simulink model "yidongshi"  (R2025b)
settings: Solver=VariableStepAuto  StartTime=0.0  StopTime=65  RelTol=1e-3
values from neighbouring files (symbols this model uses):
  ADAMS_cwd = 'D:\2022110616\yidongshi'    [Controls_Plant_1.m]
  ADAMS_exec = ''    [Controls_Plant_1.m]
  ADAMS_host = 'yangyuheng701'    [Controls_Plant_1.m]
  ADAMS_init = ''    [Controls_Plant_1.m]
  ADAMS_inputs = 'INT_YOU!INT_ZUO!INV_SHENGJIANG!INV_SHENSUO!INV_XUANZHUAN!TURN'    [Controls_Plant_1.m]
  ADAMS_outputs = 'OUT_CMX!OUT_CMY!OUT_CMZ!OUT_SHENGJIANG!OUT_SHENSUO!OUT_V_YOU!OUT_V_ZUO!OUT_XUANZHUAN!ZHUSHUI_X!ZHUSHUI_Y!ZHUSHUI_Z'    [Controls_Plant_1.m]
  ADAMS_prefix = 'Controls_Plant_1'    [Controls_Plant_1.m]
  ADAMS_static = 'no'    [Controls_Plant_1.m]
  ADAMS_sysdir = 'D:\adams\'    [Controls_Plant_1.m]
libraries: slpidlib x2
settings Model: Creator=yangy  LastModifiedBy=yangy

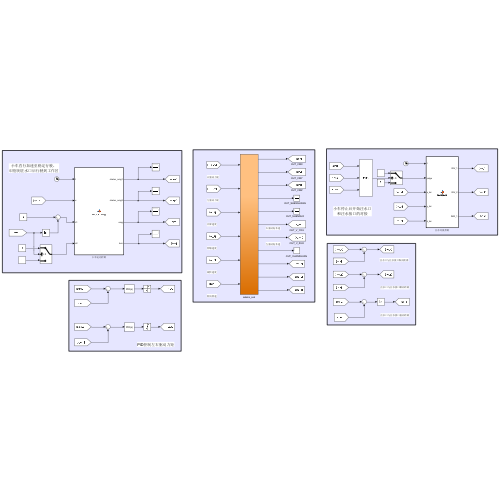
[thumbnail: Simulink's stored preview of the top-level diagram]
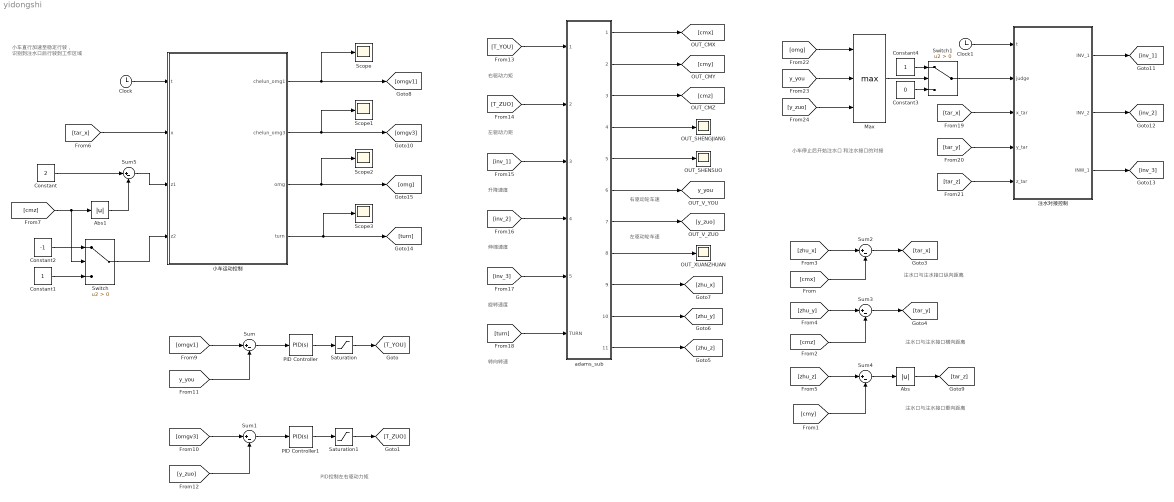
== system yidongshi ==
  note: PID控制左右驱动力矩
  note: 注水口与注水接口纵向距离
  note: 注水口与注水接口横向距离
  note: 注水口与注水接口垂向距离
  note: 小车停止后开始注水口
      | 和注水接口的对接
  note: 小车直行加速至稳定行驶，
      | 识别到注水口后行驶到工作区域
  note: 右驱动力矩
  note: 左驱动力矩
  note: 升降速度
  note: 伸缩速度
  note: 旋转速度
  note: 转向转速
  note: 右驱动轮车速
  note: 左驱动轮车速
  Abs : Abs  SaturateOnIntegerOverflow=off
  Abs1 : Abs  SaturateOnIntegerOverflow=off
  Clock : Clock
  Clock1 : Clock
  Constant : Constant  Value=2
  Constant1 : Constant
  Constant2 : Constant  Value=-1
  Constant3 : Constant  Value=0
  Constant4 : Constant
  Max : MinMax  Function=max  Inputs=3
  "OUT_SHENGJIANG     " : Scope
      settings: DataLoggingVariableName=ScopeData6
  "OUT_SHENSUO     " : Scope
      settings: DataLoggingVariableName=ScopeData7
  "OUT_XUANZHUAN " : Scope
      settings: DataLoggingVariableName=ScopeData8
  PID Controller : slpidlib/PID Controller  Controller=PID  Form=Parallel  TimeDomain=Continuous-time  UseExternalTs=off  SampleTime=-1  IntegratorMethod=Forward Euler  FilterMethod=Forward Euler  ControllerParametersSource=internal  P=1.7  I=0.1  UseKiTs=off  D=0.1  UseExternalDerivativeSource=off  N=100  UseFilter=on  TunerSelectOption=Transfer Function Based (PID Tuner App)  InitialConditionSource=internal  InitialConditionForIntegrator=0  InitialConditionForFilter=0  DifferentiatorICPrevScaledInput=0  ExternalReset=none  TrackingMode=off  Kt=1  LimitOutput=off  SatLimitsSource=internal  UpperSaturationLimit=inf  LowerSaturationLimit=-inf  LinearizeAsGain=on  AntiWindupMode=none  Kb=1  LimitIntegrator=off  UpperIntegratorSaturationLimit=inf  LowerIntegratorSaturationLimit=-inf  POutMin=[]  POutMax=[]  IOutMin=[]  IOutMax=[]  DOutMin=[]  DOutMax=[]  NOutMin=[]  NOutMax=[]  SumOutMin=[]  SumOutMax=[]  SaturationOutMin=[]  SaturationOutMax=[]  PParamMin=[]  PParamMax=[]  IParamMin=[]  IParamMax=[]  DParamMin=[]  DParamMax=[]  NParamMin=[]  NParamMax=[]  KbParamMin=[]  KbParamMax=[]  KtParamMin=[]  KtParamMax=[]  KbOutMin=[]  KbOutMax=[]  KtOutMin=[]  KtOutMax=[]  IntegratorOutMin=[]  IntegratorOutMax=[]  FilterOutMin=[]  FilterOutMax=[]  SumI1OutMin=[]  SumI1OutMax=[]  SumI2OutMin=[]  SumI2OutMax=[]  SumI3OutMin=[]  SumI3OutMax=[]  SumI4OutMin=[]  SumI4OutMax=[]  SumDOutMin=[]  SumDOutMax=[]  DifferentiatorOutMin=[]  DifferentiatorOutMax=[]  FilterDiffOutCoefMin=[]  FilterDiffOutCoefMax=[]  ReciprocalOutMin=[]  ReciprocalOutMax=[]  SumDenOutMin=[]  SumDenOutMax=[]  SumNumOutMin=[]  SumNumOutMax=[]  DivideOutMin=[]  DivideOutMax=[]  UdiffTsProdOutMin=[]  UdiffTsProdOutMax=[]  NTsProdOutMin=[]  NTsProdOutMax=[]  UintegralTsProdOutMin=[]  UintegralTsProdOutMax=[]  UngainTsProdOutMin=[]  UngainTsProdOutMax=[]  ClampingZeroOutDataTypeStr=Inherit: Inherit via back propagation  ClampingZeroOutMin=[]  ClampingZeroOutMax=[]  FilterDenConstantOutDataTypeStr=Inherit: Inherit via back propagation  FilterDenConstantOutMin=[]  FilterDenConstantOutMax=[]  PCopyOutDataTypeStr=Inherit: Inherit via back propagation  PCopyOutMin=[]  PCopyOutMax=[]  NCopyOutDataTypeStr=Inherit: Inherit via back propagation  NCopyOutMin=[]  NCopyOutMax=[]  IntegratorContinuousStateAttributes=''  IntegratorStateMustResolveToSignalObject=off  IntegratorRTWStateStorageClass=Auto  FilterContinuousStateAttributes=''  FilterStateMustResolveToSignalObject=off  FilterRTWStateStorageClass=Auto  ParallelPVariant=InternalParameters  IdealPVariant=Disabled  IVariant=InternalParameters  DVariant=InternalParameters  IntegratorVariant=Continuous  SatVariant=Disabled  AWVariant=Passthrough  PCopyVariant=Disabled  TRVariant=Disabled  FdbkBlocksVariant=Forward  IdealPFdbkVariant=Disabled  SatFdbkVariant=Disabled  DerivativeFilterVariant=ContFilter  NVariant=InternalParameters  NCopyVariant=Disabled  FilterICVariant=InternalICsFilter  IntegratorICVariant=InternalICs  ExternalResetVariant=Disabled  TRSumVariant=Passthrough  SumFdbkVariant=Disabled  SumVariant=Sum_PID  TsampFilterVariant=InternalTs  TsampNgainVariant=Passthrough  TsampIntegralVariant=Disabled_SignalSpec  ExternalSaturationOutDataTypeStr=Inherit: Same as second input  DerivativeSourceVariant=ErrorSignal  PreIntVariant=InternalPreInt
  PID Controller1 : slpidlib/PID Controller  Controller=PID  Form=Parallel  TimeDomain=Continuous-time  UseExternalTs=off  SampleTime=-1  IntegratorMethod=Forward Euler  FilterMethod=Forward Euler  ControllerParametersSource=internal  P=1.7  I=0.1  UseKiTs=off  D=0.1  UseExternalDerivativeSource=off  N=100  UseFilter=on  TunerSelectOption=Transfer Function Based (PID Tuner App)  InitialConditionSource=internal  InitialConditionForIntegrator=0  InitialConditionForFilter=0  DifferentiatorICPrevScaledInput=0  ExternalReset=none  TrackingMode=off  Kt=1  LimitOutput=off  SatLimitsSource=internal  UpperSaturationLimit=inf  LowerSaturationLimit=-inf  LinearizeAsGain=on  AntiWindupMode=none  Kb=1  LimitIntegrator=off  UpperIntegratorSaturationLimit=inf  LowerIntegratorSaturationLimit=-inf  POutMin=[]  POutMax=[]  IOutMin=[]  IOutMax=[]  DOutMin=[]  DOutMax=[]  NOutMin=[]  NOutMax=[]  SumOutMin=[]  SumOutMax=[]  SaturationOutMin=[]  SaturationOutMax=[]  PParamMin=[]  PParamMax=[]  IParamMin=[]  IParamMax=[]  DParamMin=[]  DParamMax=[]  NParamMin=[]  NParamMax=[]  KbParamMin=[]  KbParamMax=[]  KtParamMin=[]  KtParamMax=[]  KbOutMin=[]  KbOutMax=[]  KtOutMin=[]  KtOutMax=[]  IntegratorOutMin=[]  IntegratorOutMax=[]  FilterOutMin=[]  FilterOutMax=[]  SumI1OutMin=[]  SumI1OutMax=[]  SumI2OutMin=[]  SumI2OutMax=[]  SumI3OutMin=[]  SumI3OutMax=[]  SumI4OutMin=[]  SumI4OutMax=[]  SumDOutMin=[]  SumDOutMax=[]  DifferentiatorOutMin=[]  DifferentiatorOutMax=[]  FilterDiffOutCoefMin=[]  FilterDiffOutCoefMax=[]  ReciprocalOutMin=[]  ReciprocalOutMax=[]  SumDenOutMin=[]  SumDenOutMax=[]  SumNumOutMin=[]  SumNumOutMax=[]  DivideOutMin=[]  DivideOutMax=[]  UdiffTsProdOutMin=[]  UdiffTsProdOutMax=[]  NTsProdOutMin=[]  NTsProdOutMax=[]  UintegralTsProdOutMin=[]  UintegralTsProdOutMax=[]  UngainTsProdOutMin=[]  UngainTsProdOutMax=[]  ClampingZeroOutDataTypeStr=Inherit: Inherit via back propagation  ClampingZeroOutMin=[]  ClampingZeroOutMax=[]  FilterDenConstantOutDataTypeStr=Inherit: Inherit via back propagation  FilterDenConstantOutMin=[]  FilterDenConstantOutMax=[]  PCopyOutDataTypeStr=Inherit: Inherit via back propagation  PCopyOutMin=[]  PCopyOutMax=[]  NCopyOutDataTypeStr=Inherit: Inherit via back propagation  NCopyOutMin=[]  NCopyOutMax=[]  IntegratorContinuousStateAttributes=''  IntegratorStateMustResolveToSignalObject=off  IntegratorRTWStateStorageClass=Auto  FilterContinuousStateAttributes=''  FilterStateMustResolveToSignalObject=off  FilterRTWStateStorageClass=Auto  ParallelPVariant=InternalParameters  IdealPVariant=Disabled  IVariant=InternalParameters  DVariant=InternalParameters  IntegratorVariant=Continuous  SatVariant=Disabled  AWVariant=Passthrough  PCopyVariant=Disabled  TRVariant=Disabled  FdbkBlocksVariant=Forward  IdealPFdbkVariant=Disabled  SatFdbkVariant=Disabled  DerivativeFilterVariant=ContFilter  NVariant=InternalParameters  NCopyVariant=Disabled  FilterICVariant=InternalICsFilter  IntegratorICVariant=InternalICs  ExternalResetVariant=Disabled  TRSumVariant=Passthrough  SumFdbkVariant=Disabled  SumVariant=Sum_PID  TsampFilterVariant=InternalTs  TsampNgainVariant=Passthrough  TsampIntegralVariant=Disabled_SignalSpec  ExternalSaturationOutDataTypeStr=Inherit: Same as second input  DerivativeSourceVariant=ErrorSignal  PreIntVariant=InternalPreInt
  Saturation : Saturate  UpperLimit=100  LowerLimit=-100
  Saturation1 : Saturate  UpperLimit=100  LowerLimit=-100
  Scope{,1..3} (4 alike) : Scope
      Scope settings: DataLoggingVariableName=ScopeData11
      Scope2 settings: DataLoggingVariableName=ScopeData2
  Sum{,1..5} (6 alike) : Sum  Inputs=|+-
  Switch : Switch  Criteria=u2 > Threshold  SaturateOnIntegerOverflow=off  InputSameDT=off
  Switch1 : Switch  Criteria=u2 > Threshold  SaturateOnIntegerOverflow=off  InputSameDT=off
  adams_sub : Subsystem
  小车运动控制 : MATLAB Function  TreatAsAtomicUnit=on
  注水对接控制 : MATLAB Function  TreatAsAtomicUnit=on
  tag scope: y_you=global
  wires:
  Clock/1 -> 小车运动控制/1(t)
  小车运动控制/1(chelun_omg1) -> Scope/1, [omgv1]
  小车运动控制/2(chelun_omg3) -> Scope1/1, [omgv3]
  Sum/1 -> PID Controller/1
  PID Controller/1 -> Saturation/1
  Saturation/1 -> [T_YOU]
  PID Controller1/1 -> Saturation1/1
  Saturation1/1 -> [T_ZUO]
  Sum1/1 -> PID Controller1/1
  [zhu_x] -> Sum2/1
  [cmx] -> Sum2/2
  [zhu_y] -> Sum3/1
  [cmz] -> Sum3/2
  [zhu_z] -> Sum4/1
  [cmy] -> Sum4/2
  Sum4/1 -> Abs/1
  Sum2/1 -> [tar_x]
  Sum3/1 -> [tar_y]
  Abs/1 -> [tar_z]
  [tar_x] -> 小车运动控制/2(x)
  Constant/1 -> Sum5/1
  Abs1/1 -> Sum5/2
  Sum5/1 -> 小车运动控制/3(z1)
  Constant2/1 -> Switch/1
  Constant1/1 -> Switch/3
  Switch/1 -> 小车运动控制/4(z2)
  [omgv1] -> Sum/1
  [y_you] -> Sum/2
  [omgv3] -> Sum1/1
  [y_zuo] -> Sum1/2
  小车运动控制/3(omg) -> Scope2/1, [omg]
  [cmz] -> Abs1/1, Switch/2
  小车运动控制/4(turn) -> Scope3/1, [turn]
  Constant3/1 -> Switch1/3
  [T_YOU] -> adams_sub/1("INT_YOU       ")
  [T_ZUO] -> adams_sub/2("INT_ZUO       ")
  [inv_1] -> adams_sub/3(INV_SHENGJIANG)
  [inv_3] -> adams_sub/5("INV_XUANZHUAN ")
  [turn] -> adams_sub/6("TURN          ")
  adams_sub/1("OUT_CMX       ") -> [cmx]
  adams_sub/2("OUT_CMY       ") -> [cmy]
  adams_sub/3("OUT_CMZ       ") -> [cmz]
  adams_sub/4(OUT_SHENGJIANG) -> "OUT_SHENGJIANG     "/1
  adams_sub/5("OUT_SHENSUO   ") -> "OUT_SHENSUO     "/1
  adams_sub/6("OUT_V_YOU     ") -> [y_you]
  adams_sub/7("OUT_V_ZUO     ") -> [y_zuo]
  [inv_2] -> adams_sub/4("INV_SHENSUO   ")
  adams_sub/8("OUT_XUANZHUAN ") -> "OUT_XUANZHUAN "/1
  adams_sub/9("ZHUSHUI_X     ") -> [zhu_x]
  adams_sub/10("ZHUSHUI_Y     ") -> [zhu_y]
  adams_sub/11("ZHUSHUI_Z     ") -> [zhu_z]
  [omg] -> Max/1
  [y_you] -> Max/2
  [y_zuo] -> Max/3
  Constant4/1 -> Switch1/1
  Max/1 -> Switch1/2
  [tar_z] -> 注水对接控制/5(z_tar)
  [tar_y] -> 注水对接控制/4(y_tar)
  [tar_x] -> 注水对接控制/3(x_tar)
  Switch1/1 -> 注水对接控制/2(judge)
  Clock1/1 -> 注水对接控制/1(t)
  注水对接控制/1(INV_1) -> [inv_1]
  注水对接控制/2(INV_2) -> [inv_2]
  注水对接控制/3(INW_1) -> [inv_3]

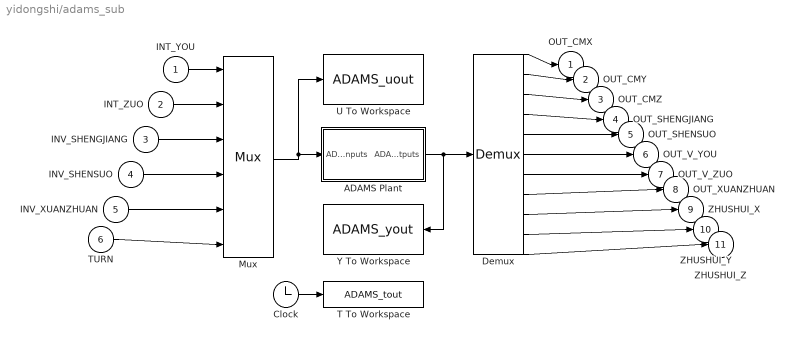
== system yidongshi/adams_sub ==
  "INT_YOU       " : Inport
  "INT_ZUO       " : Inport  Port=2
  INV_SHENGJIANG : Inport  Port=3
  "INV_SHENSUO   " : Inport  Port=4
  "INV_XUANZHUAN " : Inport  Port=5
  "TURN          " : Inport  Port=6
  ADAMS Plant : Subsystem  LoadFcn=|  InitFcn=clear mex  mask(Adams Plant){exevie=ADAMS_sysdir, nam_in=ADAMS_inputs, namout=ADAMS_outputs, nampre=ADAMS_prefix, outfil=ADAMS_prefix, exesol=ADAMS_exec, stat=ADAMS_static, inicmd=[ADAMS_init], exetyp=C++, comtyp=PIPE(DDE), workdir=ADAMS_cwd, ada_host=ADAMS_host, modani=batch, modsim=discrete, dft=no, simulink_lead_cosim=yes, pin_interp_order=0, pout_extrap_order=0, pin_extrap_order=0, pout_interp_order=0, dt_out=0.005, o_rate=1, more=off}
      | %check based on dialog box setting for when setting by popup menu                                             
      | if exist('ADAMS_solver_type')                                                                                 
      |   if strcmp(ADAMS_solver_type,'C++')                                                                          
      |     set_param(gcb,'exetyp','C++');                                                                            
      |   else                                                                                                        
      |     set_param(gcb,'exetyp','Fortran');                                                                        
      |   end                                                                                                         
      | else                                                                                                          
      |   set_param(gcb,'exetyp','C++');                                                                              
      | end                                                                                                           
      | %set the mode if using acar_solver                                                                            
      | %REQUIRED HERE BECAUSE BELOW CAUSES MDLTERMINATE TO BE CALLED 2 TIMES IN MIDDLE OF SIMULATION WHEN SET IN MASK
      |                                                                                                               
      | %enable the direct feedthrough, sim mode, anim mode parameters by default                                     
      |                                                                                                               
      | if exist('set_some_params_states')                                                                            
      |                                                                                                               
      |   set_some_params_states({'dft','modsim','modani'},{'on','on','on'},'MaskEnables',gcb)                        
      |   %turn on direct feedthrough option                                                                          
      |   set_some_params_states({'dft'},{'on'},'MaskVisibilities',gcb)                                               
      |                                                                                                               
      |  end                                                                                                          
      |                                                                                                               
      |                                                                                                               
      | if exist('ADAMS_exec')                                                                                        
      |   if and(strcmp(get_param(gcb,'exesol'),'ADAMS_exec'),strcmp(ADAMS_exec,'acar_solver'))                       
      |     %set the sim mode to discrete -- only supported mode                                                      
      |     set_param(gcb,'modsim','discrete')                                                                        
      |      %turn off direct feedthrough option                                                                      
      |      set_some_params_states({'dft'},{'off'},'MaskVisibilities',gcb)                                           
      |     %set the animation mode to batch -- only supported mode                                                   
      |     set_param(gcb,'modani','batch')                                                                           
      |     %disable the direct feedthrough, sim mode, anim mode parameters                                           
      |     set_some_params_states({'modsim','modani'},{'off','off'},'MaskEnables',gcb)                               
      |   end
      |   if and(strcmp(get_param(gcb,'exesol'),'ADAMS_exec'),strcmp(ADAMS_exec,'apre_solver'))                       
      |     %set the sim mode to discrete -- only supported mode                                                      
      |     set_param(gcb,'modsim','discrete')                                                                        
      |      %turn off direct feedthrough option                                                                      
      |      set_some_params_states({'dft'},{'off'},'MaskVisibilities',gcb)                                           
      |     %set the animation mode to batch -- only supported mode                                                   
      |     set_param(gcb,'modani','batch')                                                                           
      |     %disable the direct feedthrough, sim mode, anim mode parameters                                           
      |     set_some_params_states({'modsim','modani'},{'off','off'},'MaskEnables',gcb)                               
      |   end                                                                                                  
      | end
      mask prompts: exevie "Adams install directory"; nam_in "Adams View input names"; namout "Adams View output names"; nampre "Adams model file prefix"; outfil "Output files prefix (opt.: if blank - no output)"; exesol "User executable (opt.: if blank - use standard)"; stat "Initial static simulation flag"; inicmd "Initialization commands"; exetyp "Adams Solver type"; comtyp "Interprocess option"; workdir "Adams working directory"; ada_host "Adams host"; modani "Animation mode"; modsim "Simulation mode"; dft "Direct feedthrough"; simulink_lead_cosim "Discrete Computational Order - Simulink Leads Adams"; pin_interp_order "Plant input interpolation order"; pout_extrap_order "Plant output extrapolation order"; pin_extrap_order "Plant input extrapolation order"; pout_interp_order "Plant output interpolation order"; dt_out "Communication interval"; o_rate "Number of communications per output step"; more "More parameters"
      mask help: Simulate any Adams plant model either in Adams Solver form (.adm file) or in Adams View form (.cmd file)
      settings: OpenFcn=|
      | open_system(gcb,'mask')
      | if not(exist('set_some_params_states'))
      | 
      | warning('The script "set_some_params_states.m" cannot be found in the MATLAB PATH.  Cannot update the ADAMS Plant S-Function parameters.')
      | 
      | warning('Recommended action(optional):  run the Adams Controls .m file first to help choose the correct settings in the Adams S-Function block.')
      | 
      | end
      mask Help:
      | <html>
      | This S-Function represents the non-linear Adams Plant with the inputs sent to the Adams model <br>
      |  and the outputs generated by the Adams model.  See the Adams Controls documentation for more <br>
      | information.  This plant uses the following variables:<br>
      | <br>
      | <b>ADAMS_sysdir  :</b> Adams installation directory<br>
      | <b>ADAMS_inputs  :</b> Input variables View names vector<br>
      | <b>ADAMS_outputs :</b> Outputs variables View names vector<br>
      | <b>ADAMS_prefix  : </b>ADAMS model files prefix (.adm, .cmd); also doubles as output files prefix<br>
      | <b>ADAMS_exec :</b> Adams Solver user library or keyword (e.g., acar_solver)<br>
      | <b>ADAMS_static :</b> yes|no - initial static before Co-simulation(discrete)/Function Evaluation(continuous)<br>
      | <b>ADAMS_init :</b>Initialization commands (i.e., Adams View or Solver commands, depending on setting for Animation mode)<br>
      | <b>ADAMS_cwd : </b> Current working directory (for TCP/IP)<br>
      | <b>ADAMS_host : </b>Name of Adams server host (for TCP/IP)<br>
      | <b>ADAMS_mode :</b> Linear or non-linear (i.e., co-sim, function eval)<br>
      | <b>ADAMS_solver_type :</b>Fortran or C++ (used to set popup menu when first loaded) <br>
      | 
      | 
      | <br>
      | The following settings can be chosen:<br>
      | <br>
      | <b>Adams Solver type:</b>  Fortran or C++ (will also set ADAMS_solver_type)<br>
      | <b>Interprocess option:</b> Pipe(DDE), TCP/IP or DIRECT; TCP/IP can allow different machines run Adams and MATLAB<br>
      | <b>Animation mode:</b> batch (Solver, uses .adm) or interactive (View, uses .cmd)<br>
      | <b>Simulation mode:</b> discrete (Co-simulation) or continuous (Function Evaluation)<br>
      | <b>Discrete Computational Order - Simulink Lead Adams:</b> for discrete mode, chooses if Simulink leads the integration (yes) or lags (no);<br> if set to "no", can remove algebraic loop<br>
      | <b>Plant input interpolation order:</b> 0 = zero-order hold; 1 = linear (discrete mode only, where Simulink leads)<br>
      | <b>Plant output extrapolation order:</b> 0 = zero-order hold;1 = linear(discrete mode only, where Simulink leads)<br>
      | <b>Plant input extrapolation order:</b> 0 = zero-order hold; 1 = linear (discrete mode only, where Adams leads)<br>
      | <b>Plant output interpolation order:</b> 0 = zero-order hold;1 = linear(discrete mode only, where Adams leads)<br>
      | <b>Direct feedthrough:</b> yes|no - yes = Input directly effect output(continuous mode-only)<br>
      | <b>Communication interval:</b> Time step at which Co-simulation exchange information (e.g.,0.005); also controls <br>output for continuous mode (Function Evaluation)<br>
      | <b>Number of communications per output step: </b>Sets Adams output rate (.res, .req, .gra) integer value (default: 1)<br>
      | </html>
      mask Callback exesol:
      | if exist('set_some_params_states')
      | %enable the direct feedthrough, sim mode, anim mode parameters
      | set_some_params_states({'dft','modsim','modani'},{'on','on','on'},'MaskEnables',gcb)
      | %turn on direct feedthrough option
      | set_some_params_states({'dft'},{'on'},'MaskVisibilities',gcb)
      | end
      | 
      | if exist('ADAMS_exec')
      |   if and(strcmp(get_param(gcb,'exesol'),'ADAMS_exec'),strcmp(ADAMS_exec,'acar_solver'))
      |     %set the sim mode to discrete -- only supported mode
      |     %REMOVED:  BELOW CAUSES MDLTERMINATE TO BE CALLED 2 TIMES IN MIDDLE OF SIMULATION
      |     %Now in LoadFcn callback
      |     %set_param(gcb,'modsim','discrete')
      |      %turn off direct feedthrough option
      |     set_some_params_states({'dft'},{'off'},'MaskVisibilities',gcb)
      |     %set the animation mode to batch -- only supported mode
      |     %REMOVED:  BELOW CAUSES MDLTERMINATE TO BE CALLED 2 TIMES IN MIDDLE OF SIMULATION
      |     %Now in LoadFcn callback
      |     %set_param(gcb,'modani','batch')
      |     %disable the direct feedthrough, sim mode, anim mode parameters
      |     set_some_params_states({'modsim','modani'},{'off','off'},'MaskEnables',gcb)
      |   end
      | end
      mask TypeOptions exetyp: Fortran | C++
      mask Callback exetyp:
      | if strcmp(get_param(gcb,'exetyp'),'C++')
      |     ADAMS_solver_type='C++';
      | else
      |     ADAMS_solver_type='Fortran';
      | end
      mask TypeOptions comtyp: PIPE(DDE) | TCP/IP | DIRECT
      mask Callback comtyp:
      | if exist('set_some_params_states')
      | if strcmp(get_param(gcb,'comtyp'),'PIPE(DDE)') || strcmp(get_param(gcb,'comtyp'),'DIRECT')
      |     %turn off cwd, host options
      |     set_some_params_states({'ada_host','workdir'},{'off','off'},'MaskVisibilities',gcb)
      | else%if strcmp(get_param(gcb,'modsim'),'TCP/IP')
      |     %turn on cwd, host options
      |     set_some_params_states({'ada_host','workdir'},{'on','on'},'MaskVisibilities',gcb)
      | end
      | end
      mask TypeOptions modani: batch | interactive
      mask TypeOptions modsim: discrete | continuous
      mask Callback modsim:
      | if exist('set_some_params_states')
      | if strcmp(get_param(gcb,'modsim'),'discrete')
      |      %turn off direct feedthrough option
      |     set_some_params_states({'dft'},{'off'},'MaskVisibilities',gcb)
      |     %turn on discrete co-sim type if want to see more
      |     if strcmp(get_param(gcb,'more'),'on')
      |         set_some_params_states({'simulink_lead_cosim'},{'on'},'MaskVisibilities',gcb)
      |     end
      |     if strcmp(get_param(gcb,'simulink_lead_cosim'),'yes')
      |         %turn on interpolation/extrapolation options
      |         set_some_params_states({'pin_interp_order','pout_extrap_order',},{'on','on'},'MaskVisibilities',gcb)
      |     else
      |         set_some_params_states({'pin_extrap_order','pout_interp_order'},{'on','on'},'MaskVisibilities',gcb)
      |     end
      | else%if strcmp(get_param(gcb,'modsim'),'continuous')
      |      %turn off direct feedthrough option
      |     set_some_params_states({'dft'},{'on'},'MaskVisibilities',gcb)
      |     %turn off interpolation/extrapolation options
      |     set_some_params_states({'pin_interp_order','pout_extrap_order','pin_extrap_order','pout_interp_order','simulink_lead_cosim'},{'off','off','off','off','off'},'MaskVisibilities',gcb)
      | end
      | end
      mask TypeOptions dft: no | yes
      mask TypeOptions simulink_lead_cosim: yes | no
      mask Callback simulink_lead_cosim:
      | if exist('set_some_params_states')
      | if (strcmp(get_param(gcb,'simulink_lead_cosim'),'yes') && strcmp(get_param(gcb,'modsim'),'discrete'))
      |      %turn off unused interpolate/extrapolate options
      |     set_some_params_states({'pin_extrap_order','pout_interp_order'},{'off','off'},'MaskVisibilities',gcb)
      |     %turn on used interpolate/extrapolate options
      |     set_some_params_states({'pin_interp_order','pout_extrap_order'},{'on','on'},'MaskVisibilities',gcb)
      | elseif (strcmp(get_param(gcb,'simulink_lead_cosim'),'no') && strcmp(get_param(gcb,'modsim'),'discrete'))
      |     %turn on used interpolate/extrapolate options
      |     set_some_params_states({'pin_extrap_order','pout_interp_order'},{'on','on'},'MaskVisibilities',gcb)
      |      %turn off unused interpolate/extrapolate options
      |     set_some_params_states({'pin_interp_order','pout_extrap_order'},{'off','off'},'MaskVisibilities',gcb)
      | end
      | end
      mask TypeOptions pin_interp_order: 0 | 1
      mask TypeOptions pout_extrap_order: 0 | 1
      mask TypeOptions pin_extrap_order: 0 | 1
      mask TypeOptions pout_interp_order: 0 | 1
      mask Callback more:
      | if exist('set_some_params_states')
      | if (strcmp(get_param(gcb,'more'),'on'))
      |      %turn on infrequently used options
      |     set_some_params_states({'exevie','nam_in','namout','exesol','stat','inicmd'},{'on','on','on','on','on','on'},'MaskVisibilities',gcb)
      |     if strcmp(get_param(gcb,'modsim'),'discrete')
      |         set_some_params_states({'simulink_lead_cosim'},{'on'},'MaskVisibilities',gcb)
      |     end
      | elseif (strcmp(get_param(gcb,'more'),'off'))
      |     %turn off infrequently used options
      |     set_some_params_states({'exevie','nam_in','namout','exesol','stat','inicmd'},{'off','off','off','off','off','off'},'MaskVisibilities',gcb)
      |     if strcmp(get_param(gcb,'modsim'),'discrete')
      |         set_some_params_states({'simulink_lead_cosim'},{'off'},'MaskVisibilities',gcb)
      |     end
      | end
      | end
      mask Display: disp( 'MSC Software' )
  Clock : Clock
  Demux : Demux  Outputs=11
      settings: DisplayOption=none
  Mux : Mux  Inputs=6
  T To Workspace : ToWorkspace  VariableName=ADAMS_tout
      settings: MaxDataPoints=100000
  U To Workspace : ToWorkspace  VariableName=ADAMS_uout
      settings: MaxDataPoints=100000
  Y To Workspace : ToWorkspace  VariableName=ADAMS_yout
      settings: MaxDataPoints=100000
  "OUT_CMX       " : Outport
  "OUT_CMY       " : Outport  Port=2
  "OUT_CMZ       " : Outport  Port=3
  OUT_SHENGJIANG : Outport  Port=4
  "OUT_SHENSUO   " : Outport  Port=5
  "OUT_V_YOU     " : Outport  Port=6
  "OUT_V_ZUO     " : Outport  Port=7
  "OUT_XUANZHUAN " : Outport  Port=8
  "ZHUSHUI_X     " : Outport  Port=9
  "ZHUSHUI_Y     " : Outport  Port=10
  "ZHUSHUI_Z     " : Outport  Port=11
  wires:
  Clock/1 -> T To Workspace/1
  Mux/1 -> ADAMS Plant/1(ADAMS inputs), U To Workspace/1
  ADAMS Plant/1(ADAMS outputs) -> Demux/1, Y To Workspace/1
  Demux/1 -> "OUT_CMX       "/1
  Demux/2 -> "OUT_CMY       "/1
  Demux/3 -> "OUT_CMZ       "/1
  Demux/4 -> OUT_SHENGJIANG/1
  Demux/5 -> "OUT_SHENSUO   "/1
  Demux/6 -> "OUT_V_YOU     "/1
  Demux/7 -> "OUT_V_ZUO     "/1
  Demux/8 -> "OUT_XUANZHUAN "/1
  Demux/9 -> "ZHUSHUI_X     "/1
  Demux/10 -> "ZHUSHUI_Y     "/1
  Demux/11 -> "ZHUSHUI_Z     "/1
  "INT_YOU       "/1 -> Mux/1
  "INT_ZUO       "/1 -> Mux/2
  INV_SHENGJIANG/1 -> Mux/3
  "INV_SHENSUO   "/1 -> Mux/4
  "INV_XUANZHUAN "/1 -> Mux/5
  "TURN          "/1 -> Mux/6

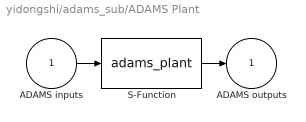
== system yidongshi/adams_sub/ADAMS Plant ==
  ADAMS inputs : Inport
  S-Function : S-Function  StopFcn=clear mex  FunctionName=adams_plant  Parameters=exevie,exesol,stat,outfil,nampre,o_rate,nam_in,namout,dft,modsim,modani,dt_out,inicmd,exetyp,comtyp,ada_host, workdir,pin_interp_order,pout_extrap_order,pin_extrap_order,pout_interp_order,simulink_lead_cosim  SFunctionDeploymentMode=off  EnableBusSupport=off
  ADAMS outputs : Outport  InitialOutput=0
  wires:
  ADAMS inputs/1 -> S-Function/1
  S-Function/1 -> ADAMS outputs/1

== matlab function yidongshi/注水对接控制 ==
  data: t input; INV_1 output; judge input; x_tar input; y_tar input; z_tar input; INV_2 output; INW_1 output
function [INV_1,INV_2,INW_1]=ZHUSHUI(t,judge,x_tar,y_tar,z_tar)
% judge: 判断是否开始对接，为0时开始对接
% X_TAR,Y_TAR,Z_TAR: 注水口在车体坐标系下坐标（x前，z右，y上）
% INV_1: 升降速度(mm/s)
% INV_2: 伸缩速度(mm/s)
% INW_1: 旋转角速度(rad/s)

% 初始与目标参数
L_init     = 300;   % 初始总长度
theta_init = 0;     % 初始旋转角(rad)
h_init     = 434;   % 初始高度(mm)

persistent active t0 theta_tar s_tar h_tar T_rot T_str T_lift T1
if isempty(active)
    active = 0;
    t0 = 0;
    theta_tar = 0; s_tar = 0; h_tar = h_init;
    T_rot = 0; T_str = 0; T_lift = 0; T1 = 0;
end

% 默认输出为0
INV_1 = 0;
INV_2 = 0;
INW_1 = 0;

% judge不为0：不对接
if judge ~= 0
    active = 0;
    t0 = 0;
    return;
end

% 开始对接
if active == 0
    active = 1;
    t0 = t;

    % 目标总长度
    L_tar = sqrt(x_tar^2 + y_tar^2);  

    % 目标旋转角
    theta_tar = atan2(y_tar, x_tar);       

    % 目标伸长量
    s_tar = L_tar - L_init;          

    % 目标高度
    h_tar = z_tar;                        

    %设定三个自由度的恒定速度
    omega = 10*pi/180;  % rad/s
    v_s   = 50;         % mm/s
    v_h   = 40;         % mm/s

    % 计算各自所需时间
    T_rot  = abs(theta_tar - theta_init) / omega;
    T_str  = abs(s_tar) / v_s;
    T_lift = abs(h_tar - h_init) / v_h;

    % 阶段1：同时旋转+伸缩，持续时间取两者较大
    T1 = max(T_rot, T_str);
end

% 局部时间 tau（从开始对接那刻算起）
tau = t - t0;
if tau < 0
    tau = 0;
end

% 分阶段输出速度命令（对应你for循环的逻辑）
omega = 10*pi/180;  % rad/s
v_s   = 50;         % mm/s
v_h   = 40;         % mm/s

if tau <= T1
    % 阶段1：同时旋转+伸缩；高度保持不动

    % 旋转：直到达到theta_tar为止（对应你dtheta判断）
    dtheta = omega * tau;
    if abs(dtheta) >= abs(theta_tar - theta_init)
        INW_1 = 0;
    else
        INW_1 = sign(theta_tar - theta_init) * omega;
    end

    % 伸缩：直到达到s_tar为止（对应你ds判断）
    ds = v_s * tau;
    if abs(ds) >= abs(s_tar)
        INV_2 = 0;
    else
        INV_2 = sign(s_tar) * v_s;
    end

    INV_1 = 0;

else
    % 阶段2：仅升降（旋转与伸缩已保持在目标值）

    INW_1 = 0;
    INV_2 = 0;

    dh = v_h * (tau - T1);
    if abs(dh) >= abs(h_tar - h_init)
        INV_1 = 0;
        % 到这里对接动作完成
    else
        INV_1 = sign(h_tar - h_init) * v_h;
    end
end

end

== matlab function yidongshi/小车运动控制 ==
  data: t input; chelun_omg1 output; x input; z1 input; z2 input; chelun_omg3 output; omg output; turn output
%% 定义期望的车轮转速曲线
function [chelun_omg1,chelun_omg3,omg,turn]=chelun_omg(t,x,z1,z2)
% t: 时间
% x: 注水口与车体的x差值
% z1: 当小车快撞上列车时紧急制动
% z2: 转向方向常数：+1=左转，-1=右转
% chelun_omg1: 左轮期望角速度
% chelun_omg3: 右轮期望角速度

% 参数
r       = 0.12;   % 轮半径(m)
v_go    = 0.5;    % 直行速度(m/s)
omg=1;
L = 0.3904;      % 左右驱动轮中心距
l = 0.66929;      % 前后轴距
rp = 0.01965;      % 小齿轮分度圆半径
la = 0.05164;      % 转向臂有效长度
eta = 0.85;      % 传动效率
%%   程序开始

persistent turning t0
if isempty(turning)
    turning = false;                        %转向是否开始
    t0 = 0;                                 %转向开始时间
end

if z1 <=0.1                                 %快要撞上，紧急制动
    turning = false;
    t0 = 0;
    vL = 0;
    vR = 0;
end
if x > 5.5                                  %没有开始转向
    turning = false;
    t0 = 0;
    vL = v_go;
    vR = v_go;
    turn = 0;

elseif x >= 0.25                             % 0.25 < x <= 5.5：转向
    if ~turning
        turning = true;                     % 第一次进入转向区间，锁存起始时刻
        t0 = t;
    end
    tau = t - t0;                           % 局部时间(从进入转向区间那一刻开始算)

    % 差速调整系数
    V=4;
    % 转弯维持时间半周期时间，即2*T完成一个转弯
    T=3.7;
    if z2 == 1
       vL=(stepfcn(tau,0,0,2,-2)+stepfcn(tau,7,0,7+T,-V) ...
           +stepfcn(tau,7+T,0,7+2*T,V)+stepfcn(tau,12+2*T,0,12+3*T,V) ...
           +stepfcn(tau,12+3*T,0,12+4*T,-V)+stepfcn(tau,12+4*T,0,13+4*T,2))*v_go;
       vR=(stepfcn(tau,0,0,2,-2)+stepfcn(tau,7,0,7+T,+V) ...
           +stepfcn(tau,7+T,0,7+2*T,-V)+stepfcn(tau,12+2*T,0,12+3*T,-V) ...
           +stepfcn(tau,12+3*T,0,12+4*T,V)+stepfcn(tau,12+4*T,0,13+4*T,2))*v_go;
    end 
    if z2 == -1
       vR=(stepfcn(tau,0,0,2,-2)+stepfcn(tau,7,0,7+T,-V) ...
           +stepfcn(tau,7+T,0,7+2*T,V)+stepfcn(tau,12+2*T,0,12+3*T,V) ...
           +stepfcn(tau,12+3*T,0,12+4*T,-V)+stepfcn(tau,12+4*T,0,13+4*T,2))*v_go;
       vL=(stepfcn(tau,0,0,2,-2)+stepfcn(tau,7,0,7+T,+V) ...
           +stepfcn(tau,7+T,0,7+2*T,-V)+stepfcn(tau,12+2*T,0,12+3*T,-V) ...
           +stepfcn(tau,12+3*T,0,12+4*T,V)+stepfcn(tau,12+4*T,0,13+4*T,2))*v_go;
    end 


   % 左右驱动轮角速度
    wL = vL / r;
    wR = vR / r;

    % 底盘线速度与角速度
    v = r/2 * (wR + wL);
    w = r/L * (wR - wL);

    % 瞬时转弯半径
    R = v / w;

    % 前轮等效转向角
    delta = atan(l / R);
    s=la*delta;
    turn = z2*s/rp;

% 开始停车制动
    elseif x<0.25
           turning = false;
           t0 = 0;
           vL = 0;
           vR = 0;
           omg=0;
           turn=0;
end


% 轮角速度
chelun_omg1 = vL/r;   % 左轮(rad/s)
chelun_omg3 = vR/r;   % 右轮(rad/s)

end


%% 子函数
function y=stepfcn(t,t1,y1,t2,y2)
y=0;
if t<t1
    y=y1;
end
if t>t2
    y=y2;
end
if (t>=t1)&&(t<=t2)
    dt=(t-t1)/(t2-t1);
    y=y1-(y1-y2)*dt^2*(3-2*dt);
end
end
